simulink model "model"  (R2022a)
settings: Solver=FixedStepAuto  StartTime=0.0  StopTime=10.0  FixedStep=0.0001  RelTol=1e-3
undefined symbols (not defined in the file): ic, K1_, K2_, T
settings Model: Creator=Egor  LastModifiedBy=P1oruN7
settings DebuggingCC: UnconnectedInputMsg=warning  UnconnectedOutputMsg=warning  UnconnectedLineMsg=warning
settings RTWCC: DLArmComputeVersion=19.05

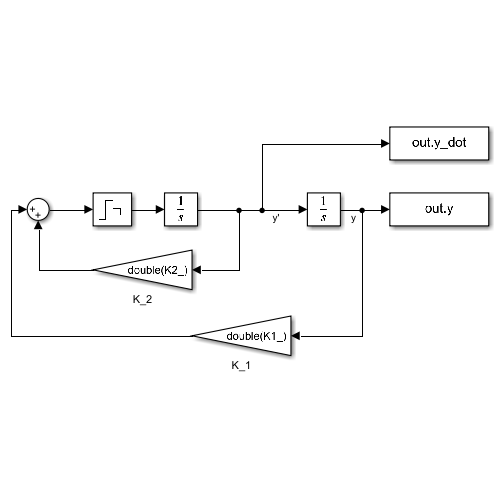
[thumbnail: Simulink's stored preview of the top-level diagram]
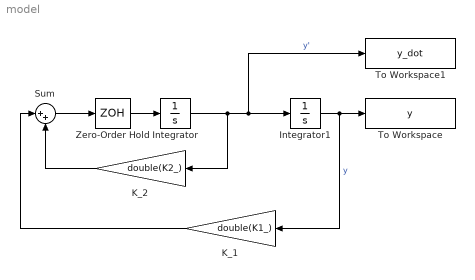
== system model ==
  Integrator : Integrator
  Integrator1 : Integrator  InitialCondition=ic
  K_1 : Gain  Gain=double(K1_)
  K_2 : Gain  Gain=double(K2_)
  Sum : Sum  Inputs=|++
  To Workspace : ToWorkspace  VariableName=y  SaveFormat=Timeseries  SampleTime=-1
  To Workspace1 : ToWorkspace  VariableName=y_dot  SaveFormat=Timeseries  SampleTime=-1
  Zero-Order Hold : ZeroOrderHold  SampleTime=T
  wires:
  Zero-Order Hold/1 -> Integrator/1
  Integrator/1 -> K_2/1, To Workspace1/1, Integrator1/1  "y'"
  Integrator1/1 -> To Workspace/1, K_1/1  "y"
  Sum/1 -> Zero-Order Hold/1
  K_1/1 -> Sum/1
  K_2/1 -> Sum/2
